simulink model "ej3"  (R2023a)
settings: Solver=VariableStepAuto  StartTime=0.0  StopTime=300  MaxStep=1e-4  RelTol=1e-3
libraries: SignalEditorBlockLib x2
settings Model: Creator=Juan  LastModifiedBy=Juan

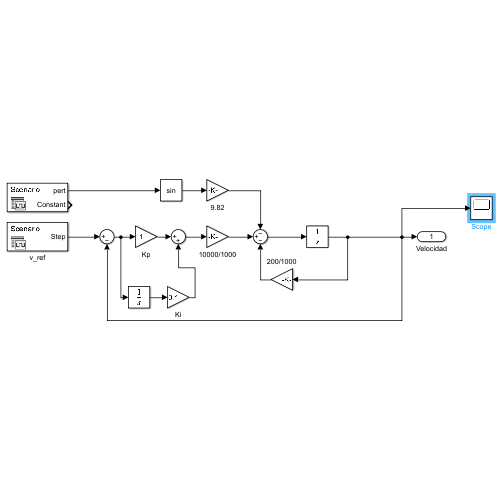
[thumbnail: Simulink's stored preview of the top-level diagram]
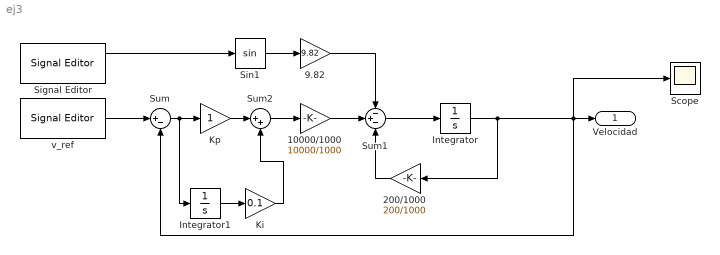
== system ej3 ==
  10000/1000 : Gain  Gain=10000/1000
  200/1000 : Gain  Gain=200/1000
  9.82 : Gain  Gain=9.82
  Integrator : Integrator  InitialCondition=25
  Integrator1 : Integrator
  Ki : Gain  Gain=0.1
  Kp : Gain
  Scope : Scope
  Signal Editor : SignalEditorBlockLib/Signal Editor  FileName=perturbn.mat  ActiveScenario=Scenario  ActiveSignal=pert  IsBus=off  OutputBusObjectStr=Bus: BusObject  SampleTime=0  Interpolate=off  ZeroCross=off  OutputAfterFinalValue=Setting to zero  Unit=inherit  PreserveSignalName=on  ApplySigPropsToAllScenarios=on
  Sin1 : Trigonometry
  Sum : Sum  Inputs=|+-
  Sum1 : Sum  Inputs=-+-
  Sum2 : Sum  Inputs=|++
  v_ref : SignalEditorBlockLib/Signal Editor  FileName=v_ref.mat  ActiveScenario=Scenario  ActiveSignal=Step  IsBus=off  OutputBusObjectStr=Bus: BusObject  SampleTime=0  Interpolate=off  ZeroCross=off  OutputAfterFinalValue=Setting to zero  Unit=inherit  PreserveSignalName=on  ApplySigPropsToAllScenarios=on
  Velocidad : Outport
  wires:
  Signal Editor/1 -> Sin1/1
  Sin1/1 -> 9.82/1
  9.82/1 -> Sum1/1
  200/1000/1 -> Sum1/3
  Sum1/1 -> Integrator/1
  Integrator/1 -> 200/1000/1, Sum/2, Scope/1, Velocidad/1
  Sum/1 -> Integrator1/1, Kp/1
  10000/1000/1 -> Sum1/2
  v_ref/1 -> Sum/1
  Sum2/1 -> 10000/1000/1
  Kp/1 -> Sum2/1
  Ki/1 -> Sum2/2
  Integrator1/1 -> Ki/1
